simulink model "doc_lmseq"  (Simulink 6.0)
settings: Solver=ode45  StartTime=0.0  StopTime=inf  RelTol=1e-3
undefined symbols (not defined in the file): qammod, slcm
libraries: commsink2 x2, commchan2 x1, dsparch4 x1, commeq2 x1, commrandsrc2 x1, commdigbbndam2 x1, dspmtrx3 x1
settings Model: Creator=agaltman  LastModifiedBy=ysong  ExtModeAutoUpdateStatusClock=off  ProdHWDeviceType=Specified
settings DataIOCC: SignalLoggingName=logsOut
settings DebuggingCC: CheckExecutionContextPreStartOutputMsg=on  CheckExecutionContextRuntimeOutputMsg=on  SolverPrmCheckMsg=none  InheritedTsInSrcMsg=none
settings HardwareCC: ProdHWDeviceType=Specified
settings ModelReferenceCC: UpdateModelReferenceTargets=IfOutOfDate
settings CodeAppCC: MangleLength=5
settings GRTTargetCC: LifeSpan=inf
settings SFSimCC: SFSimApplyToAllLibs=on  SFSimBuildMode=Incremental

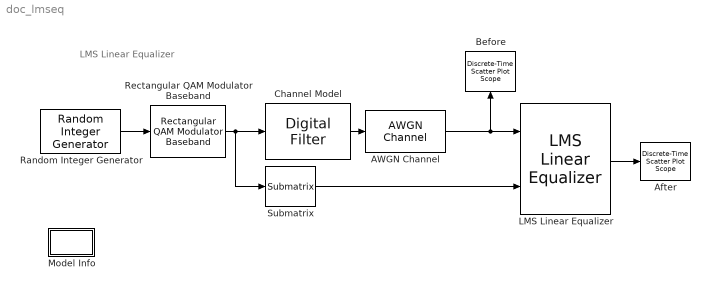
== system doc_lmseq ==
  note: LMS Linear Equalizer
  AWGN Channel : commchan2/AWGN Channel  seed=67  noiseMode="Signal to noise ratio  (SNR)"  EbNodB=10  EsNodB=10  SNRdB=40  bitsPerSym=1  Ps=1  Tsym=1  variance=1
  After : commsink2/Discrete-Time Scatter Plot Scope  Tag=ScatterPlot  sampPerSymb=1  offsetEye=0  numTraces=400  numNewFrames=10  LineMarkers=.  LineColors=b  fading=on  render=on  AxisGrid=on  xMin=-1.5  xMax=1.5  yMin=-1.5  yMax=1.5  inphaseLabel=In-phase Amplitude  quadratureLabel=Quadrature Amplitude  openScopeAtSimStart=on  FrameNumber=off  FigPos=[420 374 400 400]  figTitle=Scatter Plot  numLinesMax=8  block_type_=scatter
  Before : commsink2/Discrete-Time Scatter Plot Scope  Tag=ScatterPlot  Orientation=up  sampPerSymb=1  offsetEye=0  numTraces=400  numNewFrames=10  LineMarkers=.  LineColors=b  fading=on  render=on  AxisGrid=on  xMin=-1.5  xMax=1.5  yMin=-1.5  yMax=1.5  inphaseLabel=In-phase Amplitude  quadratureLabel=Quadrature Amplitude  openScopeAtSimStart=on  FrameNumber=off  FigPos=[10 374 400 400]  figTitle=Scatter Plot  numLinesMax=8  block_type_=scatter
  Channel Model : dsparch4/Digital Filter  TypePopup=FIR (all zeros)  IIRFiltStruct=Direct form I transposed  AllPoleFiltStruct=Direct form transposed  FIRFiltStruct=Direct form transposed  CoeffSource=Specify via dialog  NumCoeffs=[1 -.3 .1 .2j]  DenCoeffs=[1 0.1]  BiQuadCoeffs=[1 0.3 0.4 1 0.1 0.2]  LatticeCoeffs=[0.2 0.4]  denIgnore=on  FiltPerSampPopup=One filter per frame  IC=0  ICnum=0  ICden=0  roundingMode=Floor  overflowMode=off
  LMS Linear Equalizer : commeq2/LMS Linear  Equalizer  nTaps=6  nSamp=1  sigConst=qammod([0:15],16)  delay=2  stepSize=0.01  leakage=1  initWeights=0  mode=off  outErr=off  outWeights=off
  Model Info : Subsystem  LoadFcn=slcm LoadBlock;  InitFcn=slcm('UpdateAllCMBlocksInThisModelInit')  EnableExecutionContextPropagation=on  mask(CMBlock){InitialSaveTempField=, InitialBlockCM=None, BlockCM=None, Frame=on, SaveTempField=, DisplayStringWithTags=Info, MaskDisplayString=Info, HorizontalTextAlignment=Center, LeftAlignmentValue=0.5, SourceBlockDiagram=doc_lmseq, TagMaxNumber=20, CMTag1=, CMTag2=, CMTag3=, CMTag4=, CMTag5=, CMTag6=, CMTag7=, CMTag8=, CMTag9=, CMTag10=, CMTag11=, CMTag12=, CMTag13=, CMTag14=, CMTag15=, CMTag16=, CMTag17=, CMTag18=, CMTag19=, CMTag20=}
      mask help: This block allows revision control information to be displayed within the model.
      settings: CopyFcn=slcm CopyBlock;  DeleteFcn=slcm Cancel;  PostSaveFcn=slcm('UpdateAllCMBlocksInThisModel')  NameChangeFcn=slcm Rename;  OpenFcn=commdemohelp;
      mask Display: text(str2num(LeftAlignmentValue), 0.5, MaskDisplayString, 'HorizontalAlignment', HorizontalTextAlignment)
  Random Integer Generator : commrandsrc2/Random Integer Generator  mul=16  seed=12345  Ts=1/1000  frameBased=on  sampPerFrame=1000  orient=off
  Rectangular QAM Modulator Baseband : commdigbbndam2/Rectangular QAM Modulator Baseband  M=16  InType=Integer  Enc=Binary  PowType=Average Power  MinDist=2  AvgPow=1  PeakPow=1  Ph=0  numSamp=1
  Submatrix : dspmtrx3/Submatrix  RowSpan=Range of rows  RowStartMode=First  RowStartIndex=1  RowEndMode=Index  RowEndIndex=100  ColSpan=Range of columns  ColStartMode=First  ColStartIndex=1  ColEndMode=Last  ColEndIndex=1
  wires:
  Rectangular QAM Modulator Baseband/1 -> Submatrix/1, Channel Model/1
  Random Integer Generator/1 -> Rectangular QAM Modulator Baseband/1
  Channel Model/1 -> AWGN Channel/1
  LMS Linear Equalizer/1 -> After/1
  Submatrix/1 -> LMS Linear Equalizer/2
  AWGN Channel/1 -> LMS Linear Equalizer/1, Before/1

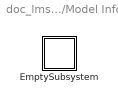
== system doc_lmseq/Model Info ==
  EmptySubsystem : Subsystem  EnableExecutionContextPropagation=on

== system doc_lmseq/Model Info/EmptySubsystem ==
